simulink model "BLDC_model2"  (R2020a)
settings: Solver=VariableStepAuto  StartTime=0.0  StopTime=10  RelTol=1e-3
InitFcn:
  | BLDC_FOC_Params
values from neighbouring files (symbols this model uses):
  J = RotorInertia_KgM2    (= 1.1e-07)    [BLDC_FOC_Params.m]    (also in systemDynamicsFunction.m = evalin('base','J'))
  Ls = PhaseSelfInductance_H    (= 0)    [BLDC_FOC_Params.m]    (also in systemDynamicsFunction.m = evalin('base','Ls'))
  PhaseTerminationIsStar = 1    [BLDC_FOC_Params.m]
  Rs = PhaseResistance_Ohm    (= 0)    [BLDC_FOC_Params.m]    (also in systemDynamicsFunction.m = evalin('base','Rs'))
  Ts = 0.0001    [BLDC_FOC_Params.m]
undefined symbols (not defined in the file or in its folder): sigbuilder_block
libraries: nesl_utility x8, ee_lib x5, eeTransforms x4, simulink x3, fl_lib x1, powerlib_meascontrol x1
settings Model: Creator=enzoe  LastModifiedBy=enzoe

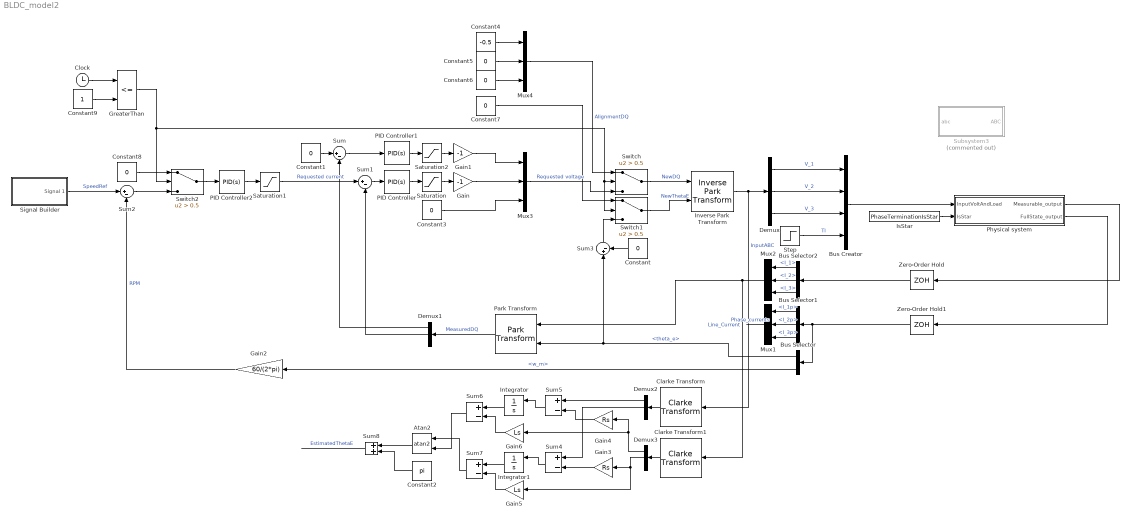
== system BLDC_model2 ==
  Atan2 : Trigonometry  Operator=atan2
  Bus Creator : BusCreator  Inputs=4
  Bus Selector : BusSelector  OutputSignals=theta_e,w_m
  Bus Selector1 : BusSelector  OutputSignals=I_1p,I_2p,I_3p
  Bus Selector2 : BusSelector  OutputSignals=I_1,I_2,I_3
  Clarke Transform : eeTransforms/Clarke Transform  PowerInvariant=off
      settings: SourceProductBaseCode=PS
  Clarke Transform1 : eeTransforms/Clarke Transform  PowerInvariant=off
      settings: SourceProductBaseCode=PS
  Clock : Clock
  Constant{,1,3,5..8} (7 alike) : Constant  Value=0
  Constant2 : Constant  Value=pi
  Constant4 : Constant  Value=-0.5
  Constant9 : Constant
  Demux{,1..3} (4 alike) : Demux  Outputs=3
  Gain : Gain  Gain=-1
  Gain1 : Gain  Gain=-1
  Gain2 : Gain  Gain=60/(2*pi)
  Gain3 : Gain  Gain=Rs
  Gain4 : Gain  Gain=Rs
  Gain5 : Gain  Gain=Ls
  Gain6 : Gain  Gain=Ls
  GreaterThan : RelationalOperator  Operator=<=  OutDataTypeStr=boolean  RndMeth=Simplest
  Integrator : Integrator  ExternalReset=rising
  Integrator1 : Integrator  ExternalReset=rising
  Inverse Park Transform : eeTransforms/Inverse Park Transform  AxisAlignment=D-axis  PowerInvariant=off
  IsStar : Constant  Value=PhaseTerminationIsStar
  Mux{1..4} (4 alike) : Mux  Inputs=3
  PID Controller : simulink/Continuous/PID Controller  Controller=PID  Form=Parallel  TimeDomain=Continuous-time  UseExternalTs=off  SampleTime=-1  IntegratorMethod=Forward Euler  FilterMethod=Forward Euler  ControllerParametersSource=internal  P=3  I=0.5  D=0  UseFilter=on  N=100  TunerSelectOption=Transfer Function Based (PID Tuner App)  InitialConditionSource=internal  InitialConditionForIntegrator=0  InitialConditionForFilter=0  DifferentiatorICPrevScaledInput=0  ExternalReset=none  TrackingMode=off  Kt=1  LimitOutput=off  UpperSaturationLimit=inf  LowerSaturationLimit=-inf  LinearizeAsGain=on  AntiWindupMode=none  Kb=1  POutMin=[]  POutMax=[]  IOutMin=[]  IOutMax=[]  DOutMin=[]  DOutMax=[]  NOutMin=[]  NOutMax=[]  SumOutMin=[]  SumOutMax=[]  SaturationOutMin=[]  SaturationOutMax=[]  PParamMin=[]  PParamMax=[]  IParamMin=[]  IParamMax=[]  DParamMin=[]  DParamMax=[]  NParamMin=[]  NParamMax=[]  KbParamMin=[]  KbParamMax=[]  KtParamMin=[]  KtParamMax=[]  KbOutMin=[]  KbOutMax=[]  KtOutMin=[]  KtOutMax=[]  IntegratorOutMin=[]  IntegratorOutMax=[]  FilterOutMin=[]  FilterOutMax=[]  SumI1OutMin=[]  SumI1OutMax=[]  SumI2OutMin=[]  SumI2OutMax=[]  SumI3OutMin=[]  SumI3OutMax=[]  SumI4OutMin=[]  SumI4OutMax=[]  SumDOutMin=[]  SumDOutMax=[]  DifferentiatorOutMin=[]  DifferentiatorOutMax=[]  FilterDiffOutCoefMin=[]  FilterDiffOutCoefMax=[]  ReciprocalOutMin=[]  ReciprocalOutMax=[]  SumDenOutMin=[]  SumDenOutMax=[]  SumNumOutMin=[]  SumNumOutMax=[]  DivideOutMin=[]  DivideOutMax=[]  UdiffTsProdOutMin=[]  UdiffTsProdOutMax=[]  NTsProdOutMin=[]  NTsProdOutMax=[]  UintegralTsProdOutMin=[]  UintegralTsProdOutMax=[]  UngainTsProdOutMin=[]  UngainTsProdOutMax=[]  IntegratorContinuousStateAttributes=''  IntegratorStateMustResolveToSignalObject=off  IntegratorRTWStateStorageClass=Auto  FilterContinuousStateAttributes=''  FilterStateMustResolveToSignalObject=off  FilterRTWStateStorageClass=Auto  ParallelPVariant=InternalParameters  IdealPVariant=Disabled  IVariant=InternalParameters  DVariant=InternalParameters  IntegratorVariant=Continuous  SatVariant=Disabled  AWVariant=Passthrough  PCopyVariant=Disabled  TRVariant=Disabled  FdbkBlocksVariant=Forward  IdealPFdbkVariant=Disabled  SatFdbkVariant=Disabled  DerivativeFilterVariant=ContFilter  NVariant=InternalParameters  NCopyVariant=Disabled  FilterICVariant=InternalICsFilter  IntegratorICVariant=InternalICs  ExternalResetVariant=Disabled  TRSumVariant=Passthrough  SumFdbkVariant=Disabled  SumVariant=Sum_PID  TsampFilterVariant=InternalTs  TsampNgainVariant=Passthrough  TsampIntegralVariant=Passthrough
  PID Controller1 : simulink/Continuous/PID Controller  Controller=PID  Form=Parallel  TimeDomain=Continuous-time  UseExternalTs=off  SampleTime=-1  IntegratorMethod=Forward Euler  FilterMethod=Forward Euler  ControllerParametersSource=internal  P=3  I=0.5  D=0  UseFilter=on  N=100  TunerSelectOption=Transfer Function Based (PID Tuner App)  InitialConditionSource=internal  InitialConditionForIntegrator=0  InitialConditionForFilter=0  DifferentiatorICPrevScaledInput=0  ExternalReset=none  TrackingMode=off  Kt=1  LimitOutput=off  UpperSaturationLimit=inf  LowerSaturationLimit=-inf  LinearizeAsGain=on  AntiWindupMode=none  Kb=1  POutMin=[]  POutMax=[]  IOutMin=[]  IOutMax=[]  DOutMin=[]  DOutMax=[]  NOutMin=[]  NOutMax=[]  SumOutMin=[]  SumOutMax=[]  SaturationOutMin=[]  SaturationOutMax=[]  PParamMin=[]  PParamMax=[]  IParamMin=[]  IParamMax=[]  DParamMin=[]  DParamMax=[]  NParamMin=[]  NParamMax=[]  KbParamMin=[]  KbParamMax=[]  KtParamMin=[]  KtParamMax=[]  KbOutMin=[]  KbOutMax=[]  KtOutMin=[]  KtOutMax=[]  IntegratorOutMin=[]  IntegratorOutMax=[]  FilterOutMin=[]  FilterOutMax=[]  SumI1OutMin=[]  SumI1OutMax=[]  SumI2OutMin=[]  SumI2OutMax=[]  SumI3OutMin=[]  SumI3OutMax=[]  SumI4OutMin=[]  SumI4OutMax=[]  SumDOutMin=[]  SumDOutMax=[]  DifferentiatorOutMin=[]  DifferentiatorOutMax=[]  FilterDiffOutCoefMin=[]  FilterDiffOutCoefMax=[]  ReciprocalOutMin=[]  ReciprocalOutMax=[]  SumDenOutMin=[]  SumDenOutMax=[]  SumNumOutMin=[]  SumNumOutMax=[]  DivideOutMin=[]  DivideOutMax=[]  UdiffTsProdOutMin=[]  UdiffTsProdOutMax=[]  NTsProdOutMin=[]  NTsProdOutMax=[]  UintegralTsProdOutMin=[]  UintegralTsProdOutMax=[]  UngainTsProdOutMin=[]  UngainTsProdOutMax=[]  IntegratorContinuousStateAttributes=''  IntegratorStateMustResolveToSignalObject=off  IntegratorRTWStateStorageClass=Auto  FilterContinuousStateAttributes=''  FilterStateMustResolveToSignalObject=off  FilterRTWStateStorageClass=Auto  ParallelPVariant=InternalParameters  IdealPVariant=Disabled  IVariant=InternalParameters  DVariant=InternalParameters  IntegratorVariant=Continuous  SatVariant=Disabled  AWVariant=Passthrough  PCopyVariant=Disabled  TRVariant=Disabled  FdbkBlocksVariant=Forward  IdealPFdbkVariant=Disabled  SatFdbkVariant=Disabled  DerivativeFilterVariant=ContFilter  NVariant=InternalParameters  NCopyVariant=Disabled  FilterICVariant=InternalICsFilter  IntegratorICVariant=InternalICs  ExternalResetVariant=Disabled  TRSumVariant=Passthrough  SumFdbkVariant=Disabled  SumVariant=Sum_PID  TsampFilterVariant=InternalTs  TsampNgainVariant=Passthrough  TsampIntegralVariant=Passthrough
  PID Controller2 : simulink/Continuous/PID Controller  Controller=PID  Form=Parallel  TimeDomain=Continuous-time  UseExternalTs=off  SampleTime=-1  IntegratorMethod=Forward Euler  FilterMethod=Forward Euler  ControllerParametersSource=internal  P=0.002  I=0.002  D=0  UseFilter=on  N=100  TunerSelectOption=Transfer Function Based (PID Tuner App)  InitialConditionSource=internal  InitialConditionForIntegrator=0  InitialConditionForFilter=0  DifferentiatorICPrevScaledInput=0  ExternalReset=none  TrackingMode=off  Kt=1  LimitOutput=off  UpperSaturationLimit=inf  LowerSaturationLimit=-inf  LinearizeAsGain=on  AntiWindupMode=none  Kb=1  POutMin=[]  POutMax=[]  IOutMin=[]  IOutMax=[]  DOutMin=[]  DOutMax=[]  NOutMin=[]  NOutMax=[]  SumOutMin=[]  SumOutMax=[]  SaturationOutMin=[]  SaturationOutMax=[]  PParamMin=[]  PParamMax=[]  IParamMin=[]  IParamMax=[]  DParamMin=[]  DParamMax=[]  NParamMin=[]  NParamMax=[]  KbParamMin=[]  KbParamMax=[]  KtParamMin=[]  KtParamMax=[]  KbOutMin=[]  KbOutMax=[]  KtOutMin=[]  KtOutMax=[]  IntegratorOutMin=[]  IntegratorOutMax=[]  FilterOutMin=[]  FilterOutMax=[]  SumI1OutMin=[]  SumI1OutMax=[]  SumI2OutMin=[]  SumI2OutMax=[]  SumI3OutMin=[]  SumI3OutMax=[]  SumI4OutMin=[]  SumI4OutMax=[]  SumDOutMin=[]  SumDOutMax=[]  DifferentiatorOutMin=[]  DifferentiatorOutMax=[]  FilterDiffOutCoefMin=[]  FilterDiffOutCoefMax=[]  ReciprocalOutMin=[]  ReciprocalOutMax=[]  SumDenOutMin=[]  SumDenOutMax=[]  SumNumOutMin=[]  SumNumOutMax=[]  DivideOutMin=[]  DivideOutMax=[]  UdiffTsProdOutMin=[]  UdiffTsProdOutMax=[]  NTsProdOutMin=[]  NTsProdOutMax=[]  UintegralTsProdOutMin=[]  UintegralTsProdOutMax=[]  UngainTsProdOutMin=[]  UngainTsProdOutMax=[]  IntegratorContinuousStateAttributes=''  IntegratorStateMustResolveToSignalObject=off  IntegratorRTWStateStorageClass=Auto  FilterContinuousStateAttributes=''  FilterStateMustResolveToSignalObject=off  FilterRTWStateStorageClass=Auto  ParallelPVariant=InternalParameters  IdealPVariant=Disabled  IVariant=InternalParameters  DVariant=InternalParameters  IntegratorVariant=Continuous  SatVariant=Disabled  AWVariant=Passthrough  PCopyVariant=Disabled  TRVariant=Disabled  FdbkBlocksVariant=Forward  IdealPFdbkVariant=Disabled  SatFdbkVariant=Disabled  DerivativeFilterVariant=ContFilter  NVariant=InternalParameters  NCopyVariant=Disabled  FilterICVariant=InternalICsFilter  IntegratorICVariant=InternalICs  ExternalResetVariant=Disabled  TRSumVariant=Passthrough  SumFdbkVariant=Disabled  SumVariant=Sum_PID  TsampFilterVariant=InternalTs  TsampNgainVariant=Passthrough  TsampIntegralVariant=Passthrough
  Park Transform : eeTransforms/Park Transform  AxisAlignment=D-axis  PowerInvariant=off
  Physical system : Subsystem
  Saturation : Saturate  UpperLimit=12  LowerLimit=-12
  Saturation1 : Saturate  UpperLimit=20  LowerLimit=-20
  Saturation2 : Saturate  UpperLimit=12  LowerLimit=-12
  Signal Builder : Subsystem  Tag=STV Subsys  LoadFcn=sigbuilder_block('load');  StartFcn=sigbuilder_block('start');  StopFcn=sigbuilder_block('stop');  ClipboardFcn=sigbuilder_block('clipboard');  mask(Sigbuilder block){tuvar=[0:10]}
      mask help: Simulink:masks:SigbuilderBlock_MD
      mask init:
      | if ~strcmp(get_param(bdroot(gcbh),'SimulationStatus'),'stopped') tuvar = sigbuilder_block('maskInit'); end
      settings: CopyFcn=sigbuilder_block('copy');  DeleteFcn=sigbuilder_block('delete');  ModelCloseFcn=sigbuilder_block('modelClose');  PreSaveFcn=sigbuilder_block('preSave');  PauseFcn=sigbuilder_block('pause');  ContinueFcn=sigbuilder_block('continue');  NameChangeFcn=sigbuilder_block('namechange');  OpenFcn=sigbuilder_block('open',[778.5 204.75 550.5 399.75 ]);  CloseFcn=sigbuilder_block('close');
      mask Display: plot(0, 0, 100, 100,[2, 2, 32, 32, 2], [68, 8, 8, 68, 68],[32, 2], [38, 38], [32, 19, 2],[53, 60, 44], [32, 17, 17, 2],[16, 16, 31, 31]);txt = getActiveGroup(gcbh);text(2, 100, txt,'verticalAlignment', 'top');
  Step : Step  Time=0  After=0  SampleTime=0
  Subsystem3 : Subsystem  Commented=on
  Sum{,1..3} (4 alike) : Sum  Inputs=|+-
  Sum{4..7} (4 alike) : Sum  Inputs=+-
  Sum8 : Sum
  Switch : Switch  Criteria=u2 > Threshold  Threshold=0.5
  Switch1 : Switch  Criteria=u2 > Threshold  Threshold=0.5
  Switch2 : Switch  Criteria=u2 > Threshold  Threshold=0.5
  Zero-Order Hold : ZeroOrderHold  SampleTime=Ts
  Zero-Order Hold1 : ZeroOrderHold  SampleTime=Ts
  wires:
  Demux/1 -> Bus Creator/1  "V_1"
  Demux/2 -> Bus Creator/2  "V_2"
  Demux/3 -> Bus Creator/3  "V_3"
  Step/1 -> Bus Creator/4  "Tl"
  Inverse Park Transform/1 -> Clarke Transform/1, Demux/1  "InputABC"
  Bus Selector1/2 -> Mux1/2  "<I_2p>"
  Bus Selector1/1 -> Mux1/1  "<I_1p>"
  Bus Selector1/3 -> Mux1/3  "<I_3p>"
  Saturation/1 -> Gain/1
  Switch/1 -> Inverse Park Transform/1  "NewDQ"
  PID Controller2/1 -> Saturation1/1
  Sum1/1 -> PID Controller/1
  Demux1/1 -> Sum/2
  Sum/1 -> PID Controller1/1
  PID Controller1/1 -> Saturation2/1
  Demux1/2 -> Sum1/2
  Constant1/1 -> Sum/1
  Signal Builder/1(Signal 1) -> Sum2/1  "SpeedRef"
  PID Controller/1 -> Saturation/1
  Constant3/1 -> Mux3/3
  Park Transform/1 -> Demux1/1  "MeasuredDQ"
  Saturation2/1 -> Gain1/1
  Bus Creator/1 -> Physical system/1(InputVoltAndLoad)
  Physical system/2(FullState_output) -> Zero-Order Hold1/1
  Physical system/1(Measurable_output) -> Zero-Order Hold/1
  Bus Selector2/1 -> Mux2/1  "<I_1>"
  Bus Selector2/2 -> Mux2/2  "<I_2>"
  Bus Selector2/3 -> Mux2/3  "<I_3>"
  Constant/1 -> Sum3/2
  Sum3/1 -> Switch1/3
  Gain2/1 -> Sum2/2  "RPM"
  Gain1/1 -> Mux3/1
  Gain/1 -> Mux3/2
  Constant4/1 -> Mux4/1
  Constant5/1 -> Mux4/2
  Constant6/1 -> Mux4/3
  Mux4/1 -> Switch/1  "AlignmentDQ"
  Constant7/1 -> Switch1/1
  Mux3/1 -> Switch/3  "Requested voltage"
  Switch1/1 -> Inverse Park Transform/2  "NewThetaE"
  Switch2/1 -> PID Controller2/1
  Sum2/1 -> Switch2/3
  Constant8/1 -> Switch2/1
  Clock/1 -> GreaterThan/1
  Constant9/1 -> GreaterThan/2
  GreaterThan/1 -> Switch1/2, Switch/2, Switch2/2
  Zero-Order Hold/1 -> Bus Selector2/1
  Zero-Order Hold1/1 -> Bus Selector/1, Bus Selector1/1
  Mux2/1 -> Clarke Transform1/1, Park Transform/1  "Line_Current"
  Mux1/1 -> ?  "Phase_currents"
  Bus Selector/2 -> Gain2/1  "<w_m>"
  Bus Selector/1 -> Sum3/1, Park Transform/2  "<theta_e>"
  IsStar/1 -> Physical system/2(IsStar)
  Saturation1/1 -> Sum1/1  "Requested current"
  Clarke Transform/1 -> Demux2/1
  Clarke Transform1/1 -> Demux3/1
  Demux3/2 -> Gain5/1, Gain3/1
  Demux3/1 -> Gain6/1, Gain4/1
  Gain3/1 -> Sum4/2
  Demux2/2 -> Sum4/1
  Sum4/1 -> Integrator1/1
  Sum5/1 -> Integrator/1
  Gain4/1 -> Sum5/2
  Demux2/1 -> Sum5/1
  Integrator/1 -> Sum6/1
  Gain6/1 -> Sum6/2
  Gain5/1 -> Sum7/2
  Integrator1/1 -> Sum7/1
  Sum7/1 -> Atan2/1
  Sum6/1 -> Atan2/2
  Atan2/1 -> Sum8/1
  Constant2/1 -> Sum8/2
  Sum8/1 -> ?  "EstimatedThetaE"

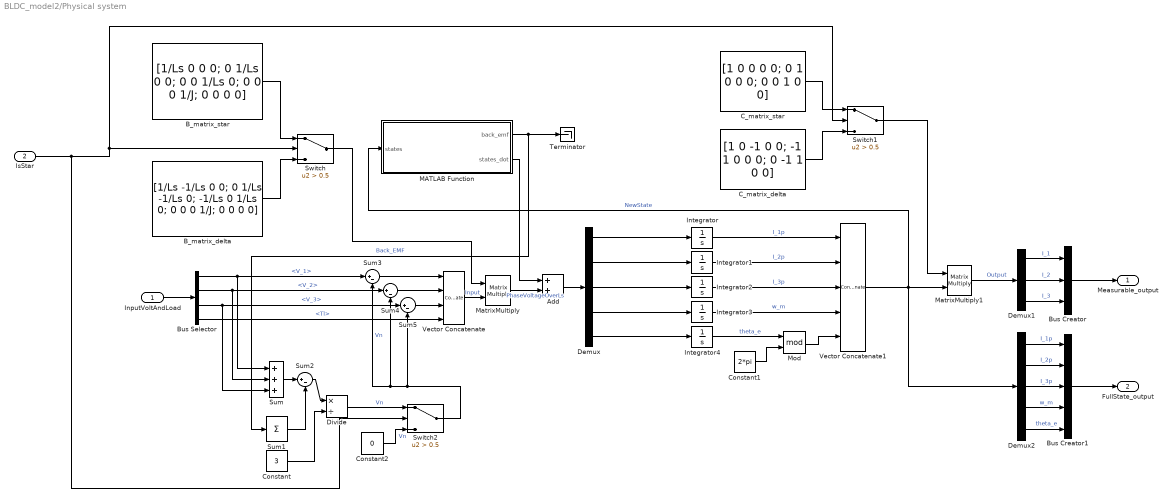
== system BLDC_model2/Physical system ==
  InputVoltAndLoad : Inport
  IsStar : Inport  Port=2
  Add : Sum
  B_matrix_delta : Constant  Value=[1/Ls -1/Ls 0 0; 0 1/Ls -1/Ls 0; -1/Ls 0 1/Ls 0; 0 0 0 1/J; 0 0 0 0]
  B_matrix_star : Constant  Value=[1/Ls 0 0 0; 0 1/Ls 0 0; 0 0 1/Ls 0; 0 0 0 1/J; 0 0 0 0]
  Bus Creator : BusCreator  Inputs=3
  Bus Creator1 : BusCreator  Inputs=5
  Bus Selector : BusSelector  OutputSignals=V_1,V_2,V_3,Tl
  C_matrix_delta : Constant  Value=[1 0 -1 0 0; -1 1 0 0 0; 0 -1 1 0 0]  VectorParams1D=off
  C_matrix_star : Constant  Value=[1 0 0 0 0; 0 1 0 0 0; 0 0 1 0 0]  VectorParams1D=off
  Constant : Constant  Value=3
  Constant1 : Constant  Value=2*pi
  Constant2 : Constant  Value=0
  Demux : Demux  Outputs=5
  Demux1 : Demux  Outputs=3
  Demux2 : Demux  Outputs=5
  Divide : Product  Inputs=*/
  Integrator{,1..4} (5 alike) : Integrator
  MATLAB Function : MATLAB Function  TreatAsAtomicUnit=on
  MatrixMultiply : Product  Multiplication=Matrix(*)
  MatrixMultiply1 : Product  Multiplication=Matrix(*)
  Mod : Math  Operator=mod  SaturateOnIntegerOverflow=on
  Sum : Sum  Inputs=+++
  Sum1 : Sum  Inputs=+
  Sum{2..5} (4 alike) : Sum  Inputs=|+-
  Switch : Switch  Criteria=u2 > Threshold  Threshold=0.5
  Switch1 : Switch  Criteria=u2 > Threshold  Threshold=0.5
  Switch2 : Switch  Criteria=u2 > Threshold  Threshold=0.5
  Terminator : Terminator
  Vector Concatenate : Concatenate  NumInputs=4  Mode=Multidimensional array
  Vector Concatenate1 : Concatenate  NumInputs=5  Mode=Multidimensional array
  Measurable_output : Outport
  FullState_output : Outport  Port=2
  wires:
  InputVoltAndLoad/1 -> Bus Selector/1
  Bus Selector/1 -> Sum3/1, Sum/1  "<V_1>"
  Bus Selector/2 -> Sum4/1, Sum/2  "<V_2>"
  Bus Selector/3 -> Sum5/1, Sum/3  "<V_3>"
  Bus Selector/4 -> Vector Concatenate/4  "<Tl>"
  Vector Concatenate/1 -> MatrixMultiply/2  "Input"
  Integrator/1 -> Vector Concatenate1/1  "I_1p"
  Integrator1/1 -> Vector Concatenate1/2  "I_2p"
  Integrator2/1 -> Vector Concatenate1/3  "I_3p"
  Integrator3/1 -> Vector Concatenate1/4  "w_m"
  Integrator4/1 -> Mod/1  "theta_e"
  MatrixMultiply/1 -> Add/2  "PhaseVoltageOverLs"
  Add/1 -> Demux/1
  Demux/1 -> Integrator/1
  Demux/2 -> Integrator1/1
  Demux/3 -> Integrator2/1
  Demux/4 -> Integrator3/1
  Demux/5 -> Integrator4/1
  MATLAB Function/2(states_dot) -> Add/1
  Vector Concatenate1/1 -> Demux2/1, MATLAB Function/1(states), MatrixMultiply1/2  "NewState"
  Constant1/1 -> Mod/2
  Mod/1 -> Vector Concatenate1/5
  Bus Creator/1 -> Measurable_output/1
  MatrixMultiply1/1 -> Demux1/1  "Output"
  Demux1/3 -> Bus Creator/3  "I_3"
  Demux1/2 -> Bus Creator/2  "I_2"
  Demux1/1 -> Bus Creator/1  "I_1"
  Bus Creator1/1 -> FullState_output/1
  Demux2/1 -> Bus Creator1/1  "I_1p"
  Demux2/2 -> Bus Creator1/2  "I_2p"
  Demux2/3 -> Bus Creator1/3  "I_3p"
  Demux2/4 -> Bus Creator1/4  "w_m"
  Demux2/5 -> Bus Creator1/5  "theta_e"
  MATLAB Function/1(back_emf) -> Sum1/1, Terminator/1  "Back_EMF"
  C_matrix_star/1 -> Switch1/1
  Sum/1 -> Sum2/1
  Sum1/1 -> Sum2/2
  Sum2/1 -> Divide/1
  Constant/1 -> Divide/2
  Switch2/1 -> Sum3/2, Sum4/2, Sum5/2  "Vn"
  B_matrix_star/1 -> Switch/1
  Sum4/1 -> Vector Concatenate/2
  Sum3/1 -> Vector Concatenate/1
  Sum5/1 -> Vector Concatenate/3
  B_matrix_delta/1 -> Switch/3
  Switch/1 -> MatrixMultiply/1
  IsStar/1 -> Switch2/2, Switch1/2, Switch/2
  C_matrix_delta/1 -> Switch1/3
  Switch1/1 -> MatrixMultiply1/1
  Constant2/1 -> Switch2/3  "Vn"
  Divide/1 -> Switch2/1  "Vn"

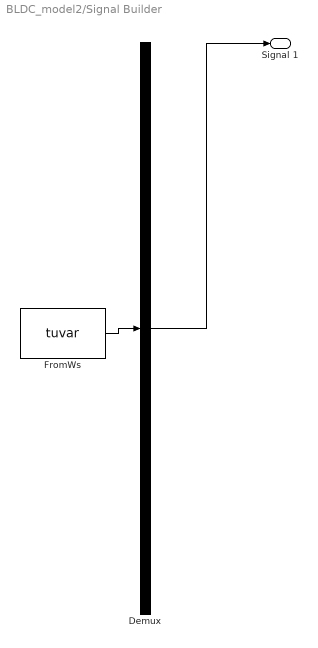
== system BLDC_model2/Signal Builder ==
  Demux : Demux  Tag=STV Demux  Outputs=1
      settings: DisplayOption=none
  FromWs : FromWorkspace  Tag=STV FromWs  VariableName=tuvar
      SigBuilderData=|
      | common.afterFinalStr = 'Extrapolate'
      | common.sampleTime = 0
      | dataSet.timeRange = [0 10]
      | dataSet.name = 'Group 1'
      | sbobj.Groups.Name = 'Group 1'
      | sbobj.Groups.Signals.Name = 'Signal 1'
      | sbobj.Groups.Signals.XData = [0 1 2 3 4 5 6 10]
      | sbobj.Groups.Signals.YData = [0 0 1000 1000 2500 2500 -1000 -1000]
  Signal 1 : Outport  Tag=STV Outport
  wires:
  Demux/1 -> Signal 1/1
  FromWs/1 -> Demux/1

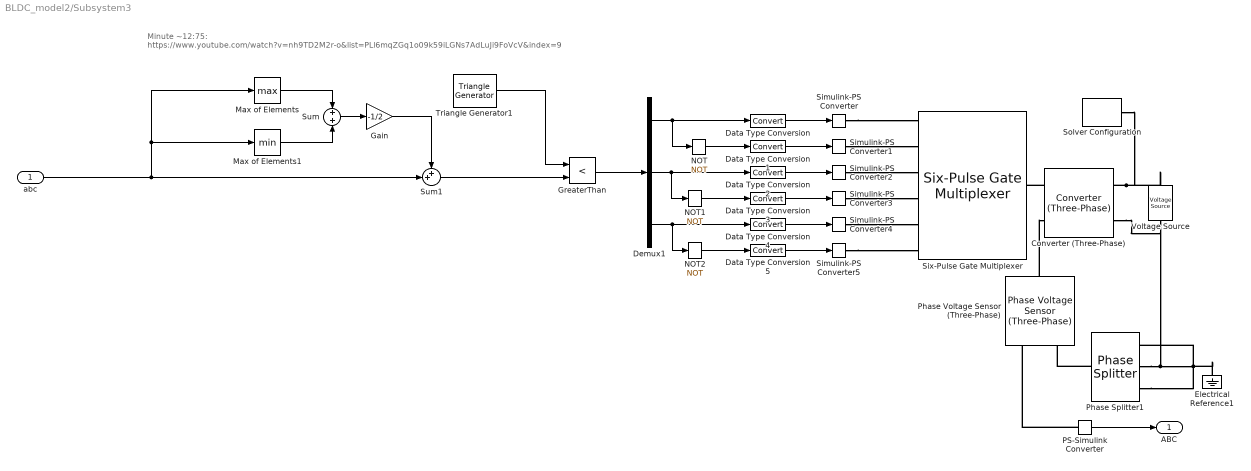
== system BLDC_model2/Subsystem3 ==
  note: Minute ~12:75:
      | https://www.youtube.com/watch?v=nh9TD2M2r-o&list=PLl6mqZGq1o09k59iLGNs7AdLuJi9FoVcV&index=9
  abc : Inport
  Converter (Three-Phase) : ee_lib/Semiconductors & Converters/Converters/Converter (Three-Phase)  device_type=ee.enum.converters.switchingdevice.ideal  Vf=0.8 V  Ron=0.001 Ohm  Rds=0.001 Ohm  Goff=1e-6 1/Ohm  Vth=6 V  Vgt=1 V  Vgt_off=-1 V  Ih=1 A  diode_param=ee.enum.converters.protectiondiode.none  diode_Vf=0.8 V  diode_Ron=0.001 Ohm  diode_Goff=1e-5 1/Ohm  diode_C=50 nF  diode_iRM=-235 A  diode_iF=300 A  diode_idot=-50 A/us  diode_trr_param=ee.enum.converters.diodetrr.trr_factor  diode_trr_factor=3  diode_trr=15 us  diode_Qrr=1500 s*uA  snubber_type=ee.enum.converters.snubber.exclude  Rs=0.1 Ohm  Cs=1e-7 F
      settings: SourceProductBaseCode=PS
  Data Type Conversion{,1..5} (6 alike) : DataTypeConversion
  Demux1 : Demux  Outputs=3
  Electrical Reference1 : fl_lib/Electrical/Electrical Elements/Electrical Reference
  Gain : Gain  Gain=-1/2
  GreaterThan : RelationalOperator  Operator=<  OutDataTypeStr=boolean  RndMeth=Simplest
  Max of Elements : MinMax  Function=max
  Max of Elements1 : MinMax
  NOT : Logic  Operator=NOT  IconShape=distinctive  AllPortsSameDT=off  OutDataTypeStr=boolean
  NOT1 : Logic  Operator=NOT  IconShape=distinctive  AllPortsSameDT=off  OutDataTypeStr=boolean
  NOT2 : Logic  Operator=NOT  IconShape=distinctive  AllPortsSameDT=off  OutDataTypeStr=boolean
  PS-Simulink Converter : nesl_utility/PS-Simulink Converter  PhysicalDomain=network_engine_domain  SubClassName=ps_output  LeftPortType=input  RightPortType=output  PseudoPeriodic=off  Frequencies=[]  Unit=inherit  AffineConversion=off
  Phase Splitter1 : ee_lib/Connectors & References/Phase Splitter
      settings: SourceProductBaseCode=PS
  Phase Voltage Sensor (Three-Phase) : ee_lib/Sensors & Transducers/Phase Voltage Sensor (Three-Phase)
      settings: SourceProductBaseCode=PS
  Simulink-PS Converter{,1..5} (6 alike) : nesl_utility/Simulink-PS Converter  PhysicalDomain=network_engine_domain  SubClassName=ps_input  LeftPortType=input  RightPortType=output  PseudoPeriodic=off  Frequencies=[]  NoiseDistribution=none  NoiseParameters=[]  Unit=1  AffineConversion=off  FilteringAndDerivatives=provide  SimscapeFilterOrder=1  InputFilterTimeConstant=0.001  UdotUserProvided=0
  Six-Pulse Gate Multiplexer : ee_lib/Semiconductors & Converters/Converters/Six-Pulse Gate Multiplexer  R=0 Ohm
      settings: SourceProductBaseCode=PS  InternalSimscapePortConfiguration="{\"Bottom\":[],\"Left\":[{\"id\":\"GaH\",\"label\":\"Ga(H)\",\"type\":\"input\"},{\"id\":\"GaL\",\"label\":\"Ga(L)\",\"type\":\"input\"},{\"id\":\"GbH\",\"label\":\"Gb(H)\",\"type\":\"input\"},{\"id\":\"GbL\",\"label\":\"Gb(L)\",\"type\":\"input\"},{\"id\":\"GcH\",\"label\":\"Gc(H)\",\"type\":\"input\"},{\"id\":\"GcL\",\"label\":\"Gc(L)\",\"type\":\"input\"}],\"Right\":[{\"id\":\"p\",\"label\":\"G\",\"type\":\"foundation.electrical.twelve_phase\"}],\"Top\":[]}"
  Solver Configuration : nesl_utility/Solver Configuration  PhysicalDomain=network_engine_domain  SubClassName=solver  LeftPortType=input  RightPortType=generic  Tones=[]  Harmonics=[]  SimulateNoise=off  Profile=off  UseLocalSampling=off  EnableSwitchedLinearOptims=on  FrequencyDomain=off  UseCCode=off  RelTol=0.001  AbsTol=1e-06  MinStep=1e-09  ToWorkspace=off  RevertToSquareIcSolve=off  NumHomotopyIterations=100  PhasorMode=off  PhasorModeNumHarmonics=1  DoDC=off  ResidualTolerance=1e-09  UseLocalSolver=on  LocalSolverChoice=NE_BACKWARD_EULER_ADVANCER  LocalSolverSampleTime=1e-4  DoFixedCost=on  MaxNonlinIter=3  MaxModeIter=2  LinearAlgebra=auto  EquationFormulation=NE_TIME_EF  DelaysMemoryBudget=1024  AutomaticFiltering=on  FilteringTimeConstant=0.001  PartitionStorageMethod=AS_NEEDED  PartitionMemoryBudget=1024  PartitionMethod=ROBUST
  Sum : Sum  Inputs=+|+
  Sum1 : Sum  Inputs=++|
  Triangle Generator1 : powerlib_meascontrol/Pulse & Signal Generators/Triangle Generator  Freq=Svpwm_freq_hz  Phase=180  Ts=0
  Voltage Source : ee_lib/Sources/Voltage Source  dc_voltage=BatteryVoltage V  ac_voltage=0 V  ac_shift=0 rad  ac_frequency=60 Hz  noise_mode=0  PSD=0 V^2/Hz  repeatability=1  auto_seed=654458608  user_seed=0  sample_time=1e-3 s  i_specify=off  i_priority=None  i=0 A  i_nominal_specify=off  i_nominal_unit=A  i_nominal_value=1  v_specify=off  v_priority=None  v=0 V  v_nominal_specify=off  v_nominal_unit=V  v_nominal_value=1
  ABC : Outport
  wires:
  abc/1 -> Sum1/2, Max of Elements1/1, Max of Elements/1
  Max of Elements1/1 -> Sum/2
  Sum/1 -> Gain/1
  Max of Elements/1 -> Sum/1
  Triangle Generator1/1 -> GreaterThan/1
  GreaterThan/1 -> Demux1/1
  NOT/1 -> Data Type Conversion1/1
  NOT1/1 -> Data Type Conversion3/1
  NOT2/1 -> Data Type Conversion5/1
  Demux1/1 -> NOT/1, Data Type Conversion/1
  Demux1/3 -> Data Type Conversion4/1, NOT2/1
  Demux1/2 -> Data Type Conversion2/1, NOT1/1
  Gain/1 -> Sum1/1
  PS-Simulink Converter/1 -> ABC/1
  Data Type Conversion/1 -> Simulink-PS Converter/1
  Data Type Conversion1/1 -> Simulink-PS Converter1/1
  Data Type Conversion2/1 -> Simulink-PS Converter2/1
  Data Type Conversion3/1 -> Simulink-PS Converter3/1
  Data Type Conversion4/1 -> Simulink-PS Converter4/1
  Data Type Conversion5/1 -> Simulink-PS Converter5/1
  Sum1/1 -> GreaterThan/2
  connections:
  Converter (Three-Phase)/RConn1 -- Voltage Source/LConn1 -- Solver Configuration/RConn1
  Simulink-PS Converter/RConn1 -- Six-Pulse Gate Multiplexer/LConn1
  Simulink-PS Converter1/RConn1 -- Six-Pulse Gate Multiplexer/LConn2
  Simulink-PS Converter2/RConn1 -- Six-Pulse Gate Multiplexer/LConn3
  Simulink-PS Converter3/RConn1 -- Six-Pulse Gate Multiplexer/LConn4
  Simulink-PS Converter4/RConn1 -- Six-Pulse Gate Multiplexer/LConn5
  Simulink-PS Converter5/RConn1 -- Six-Pulse Gate Multiplexer/LConn6
  Converter (Three-Phase)/LConn1 -- Six-Pulse Gate Multiplexer/RConn1
  Phase Voltage Sensor (Three-Phase)/LConn1 -- Converter (Three-Phase)/LConn2
  PS-Simulink Converter/LConn1 -- Phase Voltage Sensor (Three-Phase)/RConn1
  Phase Splitter1/LConn1 -- Phase Voltage Sensor (Three-Phase)/RConn2
  Electrical Reference1/LConn1 -- Phase Splitter1/RConn1 -- Phase Splitter1/RConn3 -- Phase Splitter1/RConn2 -- Voltage Source/RConn1 -- Converter (Three-Phase)/RConn2

== matlab function BLDC_model2/Physical system/MATLAB Function ==
  data: back_emf output; states input; states_dot output size=[5 1]
function [back_emf, states_dot] = SystemDynamics(states)

%#codegen
coder.extrinsic('evalin');
Rs = 0;
Rs = evalin('base','Rs');
Ls = 0;
Ls = evalin('base','Ls');
Ke = 0;
Ke = evalin('base','Ke');
Kt = 0;
Kt = evalin('base','Kt');
J = 0;
J = evalin('base','J');
B = 0;
B = evalin('base','B');
P = 0;
P = evalin('base','P');

BackEmfGenerator = @BackEmf_sinusoid;
%BackEmfGenerator = @BackEmf_Trapezoidal;

A = [-Rs/Ls 0 0 -Ke*BackEmfGenerator(states(5))/Ls 0;
    0 -Rs/Ls 0 -Ke*BackEmfGenerator(states(5) - 2*pi/3)/Ls 0;
    0 0 -Rs/Ls -Ke*BackEmfGenerator(states(5) - 4*pi/3)/Ls 0;
    Kt*BackEmfGenerator(states(5))/J Kt*BackEmfGenerator(states(5) - 2*pi/3)/J Kt*BackEmfGenerator(states(5) - 4*pi/3)/J -B/Ls 0;
    0 0 0 P 0];

back_emf = [Ke*BackEmfGenerator(states(5)) Ke*BackEmfGenerator(states(5) - 2*pi/3) Ke*BackEmfGenerator(states(5) - 4*pi/3)] * states(4);
states_dot = A*states;

end

function BackEmf = BackEmf_Trapezoidal(angle_e_rad)
    if(angle_e_rad < 0)
        angle_e_rad = 2*pi + angle_e_rad;
    end

    % Generate the waveform
    if (0 <= angle_e_rad && angle_e_rad < pi/6)
        BackEmf = angle_e_rad * 6/pi;
    elseif (pi/6 <= angle_e_rad && angle_e_rad < 5*pi/6)
        BackEmf = 1;
    elseif (5*pi/6 <= angle_e_rad && angle_e_rad < 7*pi/6)
        BackEmf = (pi - angle_e_rad) * 6/pi;
    elseif (7*pi/6 <= angle_e_rad && angle_e_rad < 11*pi/6)
        BackEmf = -1;
    elseif (11*pi/6 <= angle_e_rad && angle_e_rad < 2*pi)
        BackEmf = (angle_e_rad - 2*pi) * 6/pi;
    else
        BackEmf = 0;
    end
end

function BackEmf = BackEmf_sinusoid(angle_e_rad)
    BackEmf = sin(angle_e_rad);
end
